simulink model "impedanceControl"  (Simulink 7.9)
settings: Solver=ode3  StartTime=0.0  StopTime=inf  FixedStep=0.01  RelTol=1e-3
libraries: WBCLibrary x7, simulink x1, dspsigops x1
settings Model: Creator=daniele  LastModifiedBy=jorhabib
settings DataIOCC: SignalLoggingSaveFormat=Dataset
settings CodeAppCC: CustomSymbolStrType=$N$R$M_T
settings GRTTargetCC: CodeReplacementLibrary=C89/C90 (ANSI)

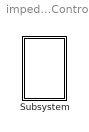
== system impedanceControl ==
  Subsystem : Subsystem  mask{robotName='icubGazeboSim', Ts=0.01, localName='dynamicBalancing'}
      mask prompts: robotName "robot name"; localName "module name"

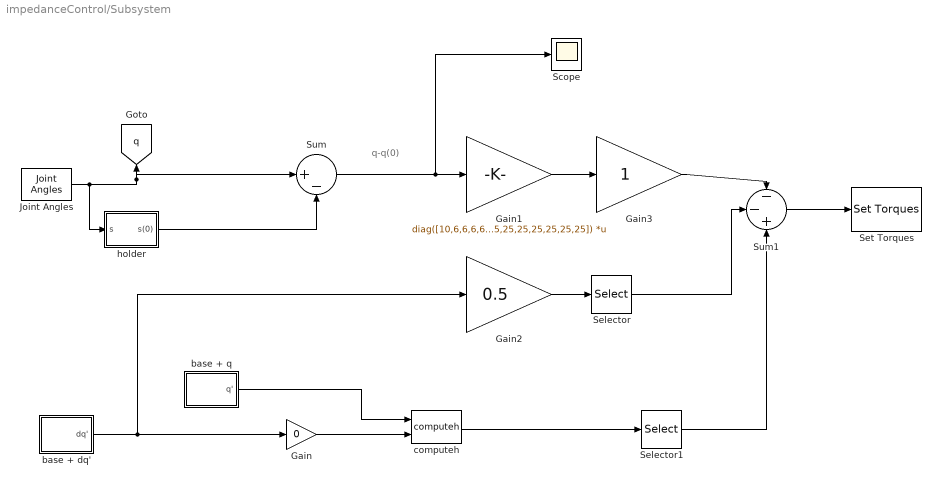
== system impedanceControl/Subsystem ==
  note: q-q(0)
  Gain : Gain  Gain=0
  Gain1 : Gain  Gain=diag([10,6,6,6,6,6,6,6,6,6,6,6,6,25,25,25,25,25,25,25,25,25,25,25,25])  Multiplication=Matrix(K*u)
  Gain2 : Gain  Gain=0.5
  Gain3 : Gain
  Joint Angles : WBCLibrary/wholeBodyStates/Joint Angles  robotName=robotName  localName=localName
  Scope : Scope
      settings: YMin=-0.3  YMax=0.6
  Selector : Selector  InputPortWidth=31  Indices=[7:31]
  Selector1 : Selector  InputPortWidth=31  Indices=[7:31]
  Set Torques : WBCLibrary/wholeBodyActuators/Set Torques  val=6  robotName=robotName  localName=localName
  Sum : Sum  Inputs=|+-
  Sum1 : Sum  Inputs=--+
  base + dq' : Subsystem
  base + q : Subsystem
  computeh : WBCLibrary/wholeBodyModel/Dynamics/computeh  val=7  robotname=robotName  localname=localName
  holder : Subsystem
  tag scope: q=global
  wires:
  base + q/1(q') -> computeh/1
  Gain/1 -> computeh/2
  holder/1(s(0)) -> Sum/2
  Sum/1 -> Scope/1, Gain1/1
  Gain2/1 -> Selector/1
  Selector/1 -> Sum1/2
  Gain1/1 -> Gain3/1
  base + dq'/1(dq') -> Gain2/1, Gain/1
  computeh/1 -> Selector1/1
  Selector1/1 -> Sum1/3
  Gain3/1 -> Sum1/1
  Joint Angles/1 -> holder/1(s), [q], Sum/1
  Sum1/1 -> Set Torques/1

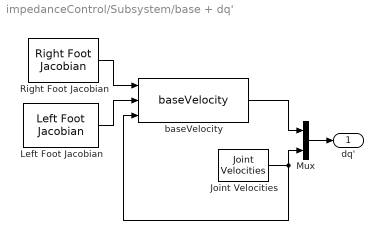
== system impedanceControl/Subsystem/base + dq' ==
  Joint Velocities : WBCLibrary/wholeBodyStates/Joint Velocities  robotName=robotName  localName=localName
  Left Foot Jacobian : WBCLibrary/wholeBodyModel/Jacobians/Left Foot Jacobian  robotName=robotName  localName=localName
  Mux : Mux  Inputs=2
  Right Foot Jacobian : WBCLibrary/wholeBodyModel/Jacobians/Right Foot Jacobian  robotName=robotName  localName=localName
  baseVelocity : WBCLibrary/Utilities/baseVelocity
  dq' : Outport
  wires:
  Left Foot Jacobian/1 -> baseVelocity/2
  Right Foot Jacobian/1 -> baseVelocity/1
  baseVelocity/1 -> Mux/1
  Joint Velocities/1 -> baseVelocity/3, Mux/2
  Mux/1 -> dq'/1

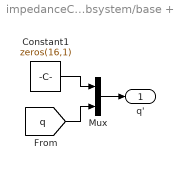
== system impedanceControl/Subsystem/base + q ==
  Constant1 : Constant  Value=zeros(16,1)
  Mux : Mux  Inputs=2
  q' : Outport
  wires:
  Mux/1 -> q'/1
  [q] -> Mux/2
  Constant1/1 -> Mux/1

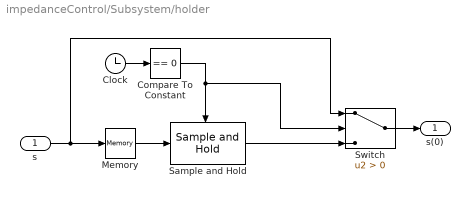
== system impedanceControl/Subsystem/holder ==
  s : Inport
  Clock : Clock
  Compare To Constant : simulink/Logic and Bit Operations/Compare To Constant  relop===  const=0  OutDataTypeStr=boolean
  Memory : Memory
  Sample and Hold : dspsigops/Sample and Hold  trig=Falling edge  initCond=0  latchinput=off
  Switch : Switch  Criteria=u2 > Threshold
  s(0) : Outport
  wires:
  s/1 -> Switch/1, Memory/1
  Clock/1 -> Compare To Constant/1
  Compare To Constant/1 -> Sample and Hold/Trigger, Switch/2
  Sample and Hold/1 -> Switch/3
  Switch/1 -> s(0)/1
  Memory/1 -> Sample and Hold/1
